simulink model "gm_Prediction_and_cost_function_FCS_MPC_6Phase_PMSM"  (R2022a)
settings: Solver=FixedStepDiscrete  StartTime=0.0  StopTime=10.0  RelTol=1e-3
undefined symbols (not defined in the file or in its folder): f_c, L_d, L_q, L_x, L_y, p, psi_pm, R_ph
libraries: hdlmdlgenlib x6
(part 1 of 2)
settings Model: Creator=Andre Merx  LastModifiedBy=Andre Merx
settings SolverCC: AlgebraicLoopSolver=TrustRegion
settings DataIOCC: LimitDataPoints=on  SaveOutput=off  SaveTime=off
settings OptimizationCC: BlockReduction=off  ConditionallyExecuteInputs=off  DefaultParameterBehavior=Inlined  LifeSpan=inf
settings DebuggingCC: AlgebraicLoopMsg=error  InheritedTsInSrcMsg=none  SingleTaskRateTransMsg=error  UnconnectedInputMsg=warning  UnconnectedOutputMsg=warning  UnconnectedLineMsg=warning  AllowSymbolicDim=off  StrictBusMsg=ErrorOnBusTreatedAsVector  SFUnexpectedBacktrackingDiag=warning  SFNoUnconditionalDefaultTransitionDiag=warning  SFExecutionAtInitializationDiag=none  SFMachineParentedDataDiag=warning  ArithmeticOperatorsInVariantConditions=warning
settings HardwareCC: ProdBitPerPointer=32  ProdBitPerSizeT=32  ProdBitPerPtrDiffT=32  ProdLargestAtomicFloat=None  ProdIntDivRoundTo=Undefined  ProdEndianess=Unspecified  ProdWordSize=32  ProdHWDeviceType=ASIC/FPGA->ASIC/FPGA  ProdEqTarget=off
settings SFSimCC: SimUseLocalCustomCode=off  CustomCodeUndefinedFunction=UseInterfaceOnly
settings RTWCC: RTWUseLocalCustomCode=off
settings CodeAppCC: StateflowObjectComments=on
settings GRTTargetCC: TargetLangStandard=C89/C90 (ANSI)
settings ConfigComp: CovScope=ReferencedModels  CovMetricSettings=dw  CovSaveCumulativeToWorkspaceVar=on  CovSaveSingleToWorkspaceVar=on  CovExternalEMLEnable=off  CovSFcnEnable=off

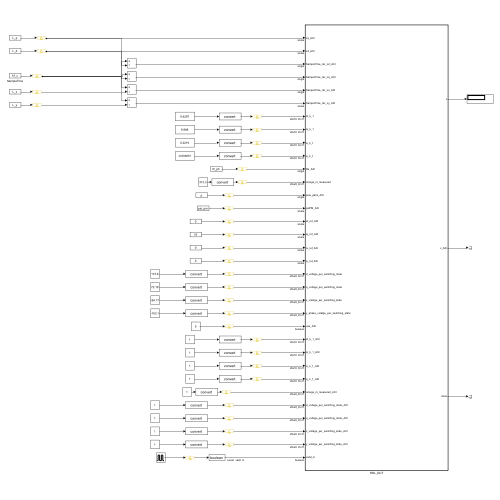
[thumbnail: Simulink's stored preview of the top-level diagram]
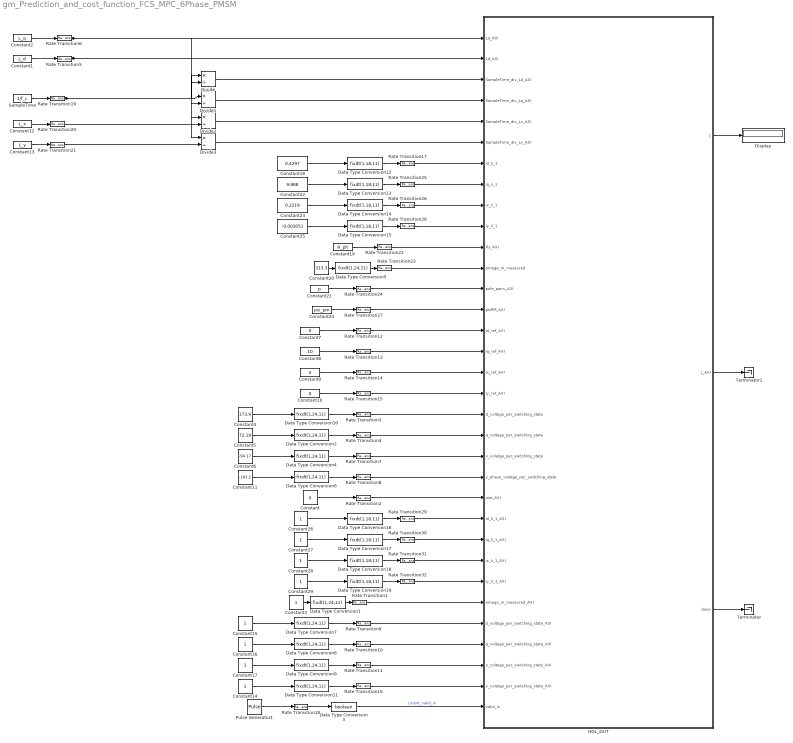
== system gm_Prediction_and_cost_function_FCS_MPC_6Phase_PMSM ==
  Constant : Constant  Value=0  OutDataTypeStr=boolean
  Constant1 : Constant  Value=L_d  OutDataTypeStr=single  SampleTime=-1
  Constant10 : Constant  Value=0  OutDataTypeStr=single  SampleTime=-1
  Constant11 : Constant  Value=-163.1
  Constant12 : Constant  Value=L_x  OutDataTypeStr=single  SampleTime=-1
  Constant13 : Constant  Value=L_y  OutDataTypeStr=single  SampleTime=-1
  Constant{3,14..17,26..29} (9 alike) : Constant
  Constant18 : Constant  Value=0.4297
  Constant19 : Constant  Value=R_ph  OutDataTypeStr=single  SampleTime=-1
  Constant2 : Constant  Value=L_q  OutDataTypeStr=single  SampleTime=-1
  Constant20 : Constant  Value=313.3
  Constant21 : Constant  Value=p  OutDataTypeStr=single  SampleTime=-1
  Constant22 : Constant  Value=9.988
  Constant23 : Constant  Value=0.2219
  Constant24 : Constant  Value=psi_pm  OutDataTypeStr=single  SampleTime=-1
  Constant25 : Constant  Value=-0.003051
  Constant4 : Constant  Value=173.9
  Constant5 : Constant  Value=72.19
  Constant6 : Constant  Value=-94.17
  Constant7 : Constant  Value=0  OutDataTypeStr=single  SampleTime=-1
  Constant8 : Constant  Value=10  OutDataTypeStr=single  SampleTime=-1
  Constant9 : Constant  Value=0  OutDataTypeStr=single  SampleTime=-1
  Data Type Conversion{1..2,4..11} (10 alike) : DataTypeConversion  OutDataTypeStr=fixdt(1,24,11)  SaturateOnIntegerOverflow=off  RndMeth=Floor
  Data Type Conversion{12..19} (8 alike) : DataTypeConversion  OutDataTypeStr=fixdt(1,18,11)  SaturateOnIntegerOverflow=off  RndMeth=Floor
  Data Type Conversion3 : DataTypeConversion  OutDataTypeStr=boolean  SaturateOnIntegerOverflow=off  RndMeth=Floor
  Display : Display
  Divide{,1..3} (4 alike) : Product  Inputs=*/  RndMeth=Zero  SaturateOnIntegerOverflow=on
  HDL_DUT : Subsystem  TreatAsAtomicUnit=on
  Pulse Generator1 : DiscretePulseGenerator  PulseType=Time based  Period=1/f_c
  Rate Transition{1..32} (32 alike) : RateTransition  OutPortSampleTime=Rt
  SampleTime : Constant  Value=1/f_c  OutDataTypeStr=single  SampleTime=-1
  Terminator : Terminator
  Terminator1 : Terminator
  wires:
  Rate Transition31/1 -> HDL_DUT/26(ix_k_1_AXI)
  Rate Transition29/1 -> HDL_DUT/24(id_k_1_AXI)
  Constant27/1 -> Data Type Conversion17/1
  Rate Transition30/1 -> HDL_DUT/25(iq_k_1_AXI)
  Data Type Conversion19/1 -> Rate Transition32/1
  Constant28/1 -> Data Type Conversion18/1
  Data Type Conversion18/1 -> Rate Transition31/1
  Data Type Conversion16/1 -> Rate Transition29/1
  Constant26/1 -> Data Type Conversion16/1
  Constant29/1 -> Data Type Conversion19/1
  Data Type Conversion17/1 -> Rate Transition30/1
  Rate Transition32/1 -> HDL_DUT/27(iy_k_1_AXI)
  Constant25/1 -> Data Type Conversion15/1
  Constant23/1 -> Data Type Conversion14/1
  Constant22/1 -> Data Type Conversion13/1
  Constant18/1 -> Data Type Conversion12/1
  Rate Transition28/1 -> HDL_DUT/10(iy_k_1)
  Data Type Conversion15/1 -> Rate Transition28/1
  Rate Transition26/1 -> HDL_DUT/9(ix_k_1)
  Data Type Conversion14/1 -> Rate Transition26/1
  Rate Transition25/1 -> HDL_DUT/8(iq_k_1)
  Data Type Conversion13/1 -> Rate Transition25/1
  Rate Transition17/1 -> HDL_DUT/7(id_k_1)
  Data Type Conversion12/1 -> Rate Transition17/1
  Rate Transition9/1 -> HDL_DUT/29(d_voltage_per_switching_state_AXI)
  Data Type Conversion7/1 -> Rate Transition9/1
  Data Type Conversion11/1 -> Rate Transition16/1
  Data Type Conversion9/1 -> Rate Transition11/1
  Data Type Conversion8/1 -> Rate Transition10/1
  Rate Transition11/1 -> HDL_DUT/31(x_voltage_per_switching_state_AXI)
  Rate Transition10/1 -> HDL_DUT/30(q_voltage_per_switching_state_AXI)
  Constant16/1 -> Data Type Conversion8/1
  Rate Transition16/1 -> HDL_DUT/32(y_volatge_per_switching_state_AXI)
  Constant14/1 -> Data Type Conversion11/1
  Constant15/1 -> Data Type Conversion7/1
  Constant17/1 -> Data Type Conversion9/1
  Constant11/1 -> Data Type Conversion6/1
  Constant6/1 -> Data Type Conversion4/1
  Constant5/1 -> Data Type Conversion2/1
  Constant4/1 -> Data Type Conversion10/1
  Rate Transition8/1 -> HDL_DUT/22(y_phase_volatge_per_switching_state)
  Data Type Conversion6/1 -> Rate Transition8/1
  Rate Transition7/1 -> HDL_DUT/21(x_volatge_per_switching_state)
  Data Type Conversion4/1 -> Rate Transition7/1
  Rate Transition4/1 -> HDL_DUT/20(q_voltage_per_switching_state)
  Data Type Conversion2/1 -> Rate Transition4/1
  Rate Transition3/1 -> HDL_DUT/19(d_voltage_per_switching_state)
  Data Type Conversion10/1 -> Rate Transition3/1
  Rate Transition2/1 -> HDL_DUT/23(use_AXI)
  Constant/1 -> Rate Transition2/1
  Rate Transition1/1 -> HDL_DUT/28(omega_m_measured_AXI)
  Data Type Conversion1/1 -> Rate Transition1/1
  Constant3/1 -> Data Type Conversion1/1
  Pulse Generator1/1 -> Rate Transition18/1
  Rate Transition18/1 -> Data Type Conversion3/1
  Data Type Conversion3/1 -> HDL_DUT/33(valid_in)  "curent_valid_in"
  HDL_DUT/1(J) -> Display/1
  HDL_DUT/2(J_AXI) -> Terminator1/1
  HDL_DUT/3(done) -> Terminator/1
  Rate Transition15/1 -> HDL_DUT/18(iy_ref_AXI)
  Rate Transition14/1 -> HDL_DUT/17(ix_ref_AXI)
  Rate Transition13/1 -> HDL_DUT/16(iq_ref_AXI)
  Rate Transition12/1 -> HDL_DUT/15(id_ref_AXI)
  Divide3/1 -> HDL_DUT/6(SampleTime_div_Ly_AXI)
  Divide2/1 -> HDL_DUT/5(SampleTime_div_Lx_AXI)
  Divide1/1 -> HDL_DUT/4(SampleTime_div_Lq_AXI)
  Divide/1 -> HDL_DUT/3(SampleTime_div_Ld_AXI)
  SampleTime/1 -> Rate Transition19/1
  Rate Transition20/1 -> Divide2/2
  Rate Transition19/1 -> Divide1/1, Divide/1, Divide2/1, Divide3/1
  Constant12/1 -> Rate Transition20/1
  Constant2/1 -> Rate Transition6/1
  Rate Transition21/1 -> Divide3/2
  Constant13/1 -> Rate Transition21/1
  Constant1/1 -> Rate Transition5/1
  Rate Transition5/1 -> Divide/2, HDL_DUT/2(Ld_AXI)
  Rate Transition6/1 -> Divide1/2, HDL_DUT/1(Lq_AXI)
  Constant19/1 -> Rate Transition22/1
  Constant20/1 -> Data Type Conversion5/1
  Rate Transition22/1 -> HDL_DUT/11(Rs_AXI)
  Rate Transition23/1 -> HDL_DUT/12(omega_m_measured)
  Constant24/1 -> Rate Transition27/1
  Constant21/1 -> Rate Transition24/1
  Data Type Conversion5/1 -> Rate Transition23/1
  Rate Transition27/1 -> HDL_DUT/14(psiPM_AXI)
  Rate Transition24/1 -> HDL_DUT/13(pole_pairs_AXI)
  Constant10/1 -> Rate Transition15/1
  Constant8/1 -> Rate Transition13/1
  Constant9/1 -> Rate Transition14/1
  Constant7/1 -> Rate Transition12/1

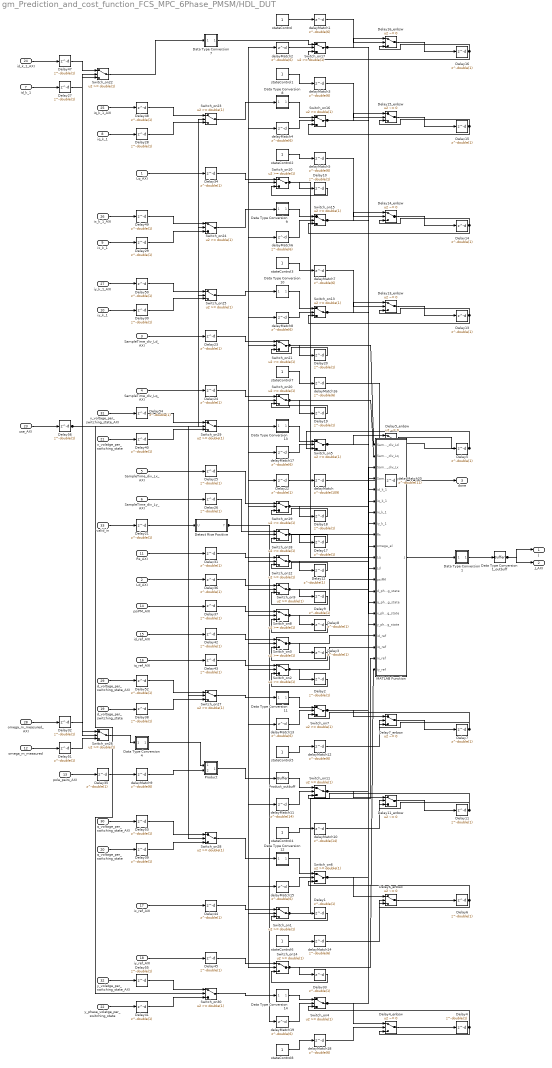
== system gm_Prediction_and_cost_function_FCS_MPC_6Phase_PMSM/HDL_DUT ==
  Lq_AXI : Inport  OutDataTypeStr=single  PortDimensions=1  SampleTime=1e-08
  Ld_AXI : Inport  Port=2  OutDataTypeStr=single  PortDimensions=1  SampleTime=1e-08
  SampleTime_div_Ld_AXI : Inport  Port=3  OutDataTypeStr=single  PortDimensions=1  SampleTime=1e-08
  SampleTime_div_Lq_AXI : Inport  Port=4  OutDataTypeStr=single  PortDimensions=1  SampleTime=1e-08
  SampleTime_div_Lx_AXI : Inport  Port=5  OutDataTypeStr=single  PortDimensions=1  SampleTime=1e-08
  SampleTime_div_Ly_AXI : Inport  Port=6  OutDataTypeStr=single  PortDimensions=1  SampleTime=1e-08
  id_k_1 : Inport  Port=7  OutDataTypeStr=fixdt(1, 18, 11)  PortDimensions=1  SampleTime=1e-08
  iq_k_1 : Inport  Port=8  OutDataTypeStr=fixdt(1, 18, 11)  PortDimensions=1  SampleTime=1e-08
  ix_k_1 : Inport  Port=9  OutDataTypeStr=fixdt(1, 18, 11)  PortDimensions=1  SampleTime=1e-08
  iy_k_1 : Inport  Port=10  OutDataTypeStr=fixdt(1, 18, 11)  PortDimensions=1  SampleTime=1e-08
  Rs_AXI : Inport  Port=11  OutDataTypeStr=single  PortDimensions=1  SampleTime=1e-08
  omega_m_measured : Inport  Port=12  OutDataTypeStr=fixdt(1, 24, 11)  PortDimensions=1  SampleTime=1e-08
  pole_pairs_AXI : Inport  Port=13  OutDataTypeStr=single  PortDimensions=1  SampleTime=1e-08
  psiPM_AXI : Inport  Port=14  OutDataTypeStr=single  PortDimensions=1  SampleTime=1e-08
  id_ref_AXI : Inport  Port=15  OutDataTypeStr=single  PortDimensions=1  SampleTime=1e-08
  iq_ref_AXI : Inport  Port=16  OutDataTypeStr=single  PortDimensions=1  SampleTime=1e-08
  ix_ref_AXI : Inport  Port=17  OutDataTypeStr=single  PortDimensions=1  SampleTime=1e-08
  iy_ref_AXI : Inport  Port=18  OutDataTypeStr=single  PortDimensions=1  SampleTime=1e-08
  d_voltage_per_switching_state : Inport  Port=19  OutDataTypeStr=fixdt(1, 24, 11)  PortDimensions=1  SampleTime=1e-08
  q_voltage_per_switching_state : Inport  Port=20  OutDataTypeStr=fixdt(1, 24, 11)  PortDimensions=1  SampleTime=1e-08
  x_volatge_per_switching_state : Inport  Port=21  OutDataTypeStr=fixdt(1, 24, 11)  PortDimensions=1  SampleTime=1e-08
  y_phase_volatge_per_switching_state : Inport  Port=22  OutDataTypeStr=fixdt(1, 24, 11)  PortDimensions=1  SampleTime=1e-08
  use_AXI : Inport  Port=23  OutDataTypeStr=boolean  PortDimensions=1  SampleTime=1e-08
  id_k_1_AXI : Inport  Port=24  OutDataTypeStr=fixdt(1, 18, 11)  PortDimensions=1  SampleTime=1e-08
  iq_k_1_AXI : Inport  Port=25  OutDataTypeStr=fixdt(1, 18, 11)  PortDimensions=1  SampleTime=1e-08
  ix_k_1_AXI : Inport  Port=26  OutDataTypeStr=fixdt(1, 18, 11)  PortDimensions=1  SampleTime=1e-08
  iy_k_1_AXI : Inport  Port=27  OutDataTypeStr=fixdt(1, 18, 11)  PortDimensions=1  SampleTime=1e-08
  omega_m_measured_AXI : Inport  Port=28  OutDataTypeStr=fixdt(1, 24, 11)  PortDimensions=1  SampleTime=1e-08
  d_voltage_per_switching_state_AXI : Inport  Port=29  OutDataTypeStr=fixdt(1, 24, 11)  PortDimensions=1  SampleTime=1e-08
  q_voltage_per_switching_state_AXI : Inport  Port=30  OutDataTypeStr=fixdt(1, 24, 11)  PortDimensions=1  SampleTime=1e-08
  x_voltage_per_switching_state_AXI : Inport  Port=31  OutDataTypeStr=fixdt(1, 24, 11)  PortDimensions=1  SampleTime=1e-08
  y_volatge_per_switching_state_AXI : Inport  Port=32  OutDataTypeStr=fixdt(1, 24, 11)  PortDimensions=1  SampleTime=1e-08
  valid_in : Inport  Port=33  OutDataTypeStr=boolean  PortDimensions=1  SampleTime=1e-08
  Data Type Conversion1 : Subsystem
      mask Display: disp('NFP\nconv');
  Data Type Conversion10 : Subsystem
      mask Display: disp('NFP\nconv');
  Data Type Conversion11 : Subsystem
      mask Display: disp('NFP\nconv');
  Data Type Conversion12 : Subsystem
      mask Display: disp('NFP\nconv');
  Data Type Conversion13 : Subsystem
      mask Display: disp('NFP\nconv');
  Data Type Conversion14 : Subsystem
      mask Display: disp('NFP\nconv');
  Data Type Conversion1_outbuff : hdlmdlgenlib/Buffer
      settings: SourceProductBaseCode=SL
  Data Type Conversion4 : Subsystem
      mask Display: disp('NFP\nconv');
  Data Type Conversion7 : Subsystem
      mask Display: disp('NFP\nconv');
  Data Type Conversion8 : Subsystem
      mask Display: disp('NFP\nconv');
  Data Type Conversion9 : Subsystem
      mask Display: disp('NFP\nconv');
  Delay{1..45,47..56} (55 alike) : Delay  DelayLength=double(1)  InitialCondition=0  SampleTime=1e-08
  Delay11_enbsw : Switch  Criteria=u2 ~= 0  Threshold=double(0)  OutDataTypeStr=single  SampleTime=1e-08  SaturateOnIntegerOverflow=off  InputSameDT=off
  Delay13_enbsw : Switch  Criteria=u2 ~= 0  Threshold=double(0)  OutDataTypeStr=single  SampleTime=1e-08  SaturateOnIntegerOverflow=off  InputSameDT=off
  Delay14_enbsw : Switch  Criteria=u2 ~= 0  Threshold=double(0)  OutDataTypeStr=single  SampleTime=1e-08  SaturateOnIntegerOverflow=off  InputSameDT=off
  Delay15_enbsw : Switch  Criteria=u2 ~= 0  Threshold=double(0)  OutDataTypeStr=single  SampleTime=1e-08  SaturateOnIntegerOverflow=off  InputSameDT=off
  Delay16_enbsw : Switch  Criteria=u2 ~= 0  Threshold=double(0)  OutDataTypeStr=single  SampleTime=1e-08  SaturateOnIntegerOverflow=off  InputSameDT=off
  Delay4_enbsw : Switch  Criteria=u2 ~= 0  Threshold=double(0)  OutDataTypeStr=single  SampleTime=1e-08  SaturateOnIntegerOverflow=off  InputSameDT=off
  Delay5_enbsw : Switch  Criteria=u2 ~= 0  Threshold=double(0)  OutDataTypeStr=single  SampleTime=1e-08  SaturateOnIntegerOverflow=off  InputSameDT=off
  Delay6_enbsw : Switch  Criteria=u2 ~= 0  Threshold=double(0)  OutDataTypeStr=single  SampleTime=1e-08  SaturateOnIntegerOverflow=off  InputSameDT=off
  Delay7_enbsw : Switch  Criteria=u2 ~= 0  Threshold=double(0)  OutDataTypeStr=single  SampleTime=1e-08  SaturateOnIntegerOverflow=off  InputSameDT=off
  Detect Rise Positive : Subsystem  mask(Detect Rise Positive){vinit=double(0), InputProcessing=Elements as channels (sample based), OutDataTypeStr=boolean}
      mask prompts: vinit "Simulink:masks:InitialCondition_MP"; InputProcessing "Simulink:masks:InputProcessing_MP"; OutDataTypeStr "Simulink:masks:OutputDataType_MP"
      mask help: Simulink:masks:DetectRisePositive_MD
      mask init:
      | InputProcessing = 'Elements as channels (sample based)';
      | OutDataTypeStr = 'boolean';
      | vinit = double(0);
      mask TypeOptions InputProcessing: Simulink:masks:ColumnsAsChannelsFrameBased | Simulink:masks:ElementsAsChannelsSampleBased
      mask TypeOptions OutDataTypeStr: Simulink:masks:uint8 | Simulink:masks:boolean
      mask Display: fprintf('U > 0\n&  NOT\nU/z > 0')
  MATLAB Function : Subsystem
  Product : Subsystem
      mask Display: disp('NFP\nmul');
  Product_outbuff : hdlmdlgenlib/Buffer
      settings: SourceProductBaseCode=SL
  Switch_on{1..21} (21 alike) : Switch  Threshold=double(1)  OutDataTypeStr=single  RndMeth=Simplest  SampleTime=1e-08  SaturateOnIntegerOverflow=off  InputSameDT=off
  Switch_on{22..25} (4 alike) : Switch  Threshold=double(1)  OutDataTypeStr=fixdt(1, 18, 11)  RndMeth=Simplest  SampleTime=1e-08  SaturateOnIntegerOverflow=off  InputSameDT=off
  Switch_on{26..30} (5 alike) : Switch  Threshold=double(1)  OutDataTypeStr=fixdt(1, 24, 11)  RndMeth=Simplest  SampleTime=1e-08  SaturateOnIntegerOverflow=off  InputSameDT=off
  delayMatch : Delay  DelayLength=double(109)  InitialCondition=0  SampleTime=1e-08
  delayMatch{1..9,12..19} (17 alike) : Delay  DelayLength=double(6)  InitialCondition=0  SampleTime=1e-08
  delayMatch10 : Delay  DelayLength=double(14)  InitialCondition=0  SampleTime=1e-08
  delayMatch11 : Delay  DelayLength=double(14)  InitialCondition=0  SampleTime=1e-08
  delayMatch20 : Delay  DelayLength=double(11)  InitialCondition=0  SampleTime=1e-08
  stateControl{,1..8} (9 alike) : Constant  OutDataTypeStr=boolean  SampleTime=1e-08
  J : Outport  SampleTime=1e-08
  J_AXI : Outport  Port=2  SampleTime=1e-08
  done : Outport  Port=3  SampleTime=1e-08
  wires:
  Lq_AXI/1 -> Delay34/1
  Ld_AXI/1 -> Delay36/1
  SampleTime_div_Ld_AXI/1 -> Delay23/1
  SampleTime_div_Lq_AXI/1 -> Delay24/1
  SampleTime_div_Lx_AXI/1 -> Delay25/1
  SampleTime_div_Ly_AXI/1 -> Delay26/1
  id_k_1/1 -> Delay27/1
  iq_k_1/1 -> Delay28/1
  ix_k_1/1 -> Delay29/1
  iy_k_1/1 -> Delay30/1
  Rs_AXI/1 -> Delay31/1
  omega_m_measured/1 -> Delay51/1
  pole_pairs_AXI/1 -> Delay35/1
  psiPM_AXI/1 -> Delay37/1
  id_ref_AXI/1 -> Delay42/1
  iq_ref_AXI/1 -> Delay43/1
  ix_ref_AXI/1 -> Delay44/1
  iy_ref_AXI/1 -> Delay45/1
  d_voltage_per_switching_state/1 -> Delay38/1
  q_voltage_per_switching_state/1 -> Delay39/1
  x_volatge_per_switching_state/1 -> Delay40/1
  y_phase_volatge_per_switching_state/1 -> Delay41/1
  use_AXI/1 -> Delay56/1
  id_k_1_AXI/1 -> Delay47/1
  iq_k_1_AXI/1 -> Delay48/1
  ix_k_1_AXI/1 -> Delay49/1
  iy_k_1_AXI/1 -> Delay50/1
  omega_m_measured_AXI/1 -> Delay32/1
  d_voltage_per_switching_state_AXI/1 -> Delay52/1
  q_voltage_per_switching_state_AXI/1 -> Delay53/1
  x_voltage_per_switching_state_AXI/1 -> Delay54/1
  y_volatge_per_switching_state_AXI/1 -> Delay55/1
  valid_in/1 -> Delay21/1
  Data Type Conversion1_outbuff/1 -> J_AXI/1, J/1
  Delay21/1 -> Detect Rise Positive/1(U)
  delayMatch20/1 -> done/1
  Delay23/1 -> Switch_on21/1
  Delay24/1 -> Switch_on20/1
  Delay25/1 -> Switch_on19/1
  Delay26/1 -> Switch_on18/1
  Delay27/1 -> Switch_on22/3
  Delay28/1 -> Switch_on23/3
  Delay29/1 -> Switch_on24/3
  Delay30/1 -> Switch_on25/3
  Delay31/1 -> Switch_on12/1
  Delay32/1 -> Switch_on26/1
  Delay34/1 -> Switch_on10/1
  delayMatch9/1 -> Product/2(In2)
  Delay36/1 -> Switch_on9/1
  Delay37/1 -> Switch_on8/1
  Delay38/1 -> Switch_on27/3
  Delay39/1 -> Switch_on28/3
  Delay40/1 -> Switch_on29/3
  Delay41/1 -> Switch_on30/3
  Delay42/1 -> Switch_on3/1
  Delay43/1 -> Switch_on2/1
  Delay44/1 -> Switch_on1/1
  Delay45/1 -> Switch_on14/1
  Delay47/1 -> Switch_on22/1
  Delay48/1 -> Switch_on23/1
  Delay49/1 -> Switch_on24/1
  Delay50/1 -> Switch_on25/1
  Delay51/1 -> Switch_on26/3
  Delay52/1 -> Switch_on27/1
  Delay53/1 -> Switch_on28/1
  Delay54/1 -> Switch_on29/1
  Delay55/1 -> Switch_on30/1
  Delay56/1 -> Switch_on30/2, Switch_on29/2, Switch_on28/2, Switch_on27/2, Switch_on26/2, Switch_on25/2, Switch_on24/2, Switch_on23/2, Switch_on22/2
  delayMatch2/1 -> Switch_on17/2
  MATLAB Function/1(J) -> Data Type Conversion1/1(In1)
  Product_outbuff/1 -> Switch_on11/1
  Switch_on1/1 -> MATLAB Function/20(ix_ref), Delay1/1
  Switch_on10/1 -> MATLAB Function/11(Lq), Delay10/1
  Switch_on12/1 -> MATLAB Function/9(Rs), Delay12/1
  Switch_on14/1 -> MATLAB Function/21(iy_ref), Delay33/1
  Switch_on18/1 -> MATLAB Function/4(SampleTime_div_Ly), Delay17/1
  Switch_on19/1 -> MATLAB Function/3(SampleTime_div_Lx), Delay18/1
  Switch_on2/1 -> MATLAB Function/19(iq_ref), Delay2/1
  Switch_on20/1 -> MATLAB Function/2(SampleTime_div_Lq), Delay19/1
  Switch_on21/1 -> MATLAB Function/1(SampleTime_div_Ld), Delay20/1
  Switch_on22/1 -> Data Type Conversion7/1(In1)
  Switch_on23/1 -> Data Type Conversion8/1(In1)
  Switch_on24/1 -> Data Type Conversion9/1(In1)
  Switch_on25/1 -> Data Type Conversion10/1(In1)
  Switch_on26/1 -> Data Type Conversion4/1(In1)
  Switch_on27/1 -> Data Type Conversion11/1(In1)
  Switch_on28/1 -> Data Type Conversion12/1(In1)
  Switch_on29/1 -> Data Type Conversion13/1(In1)
  Switch_on3/1 -> MATLAB Function/18(id_ref), Delay3/1
  Switch_on30/1 -> Data Type Conversion14/1(In1)
  Switch_on8/1 -> MATLAB Function/13(psiPM), Delay8/1
  Switch_on9/1 -> MATLAB Function/12(Ld), Delay9/1
  Delay22/1 -> delayMatch/1
  Data Type Conversion1/1(Out1) -> Data Type Conversion1_outbuff/1
  Data Type Conversion10/1(Out1) -> Switch_on13/1
  Data Type Conversion11/1(Out1) -> Switch_on7/1
  Data Type Conversion12/1(Out1) -> Switch_on6/1
  Data Type Conversion13/1(Out1) -> Switch_on5/1
  Data Type Conversion14/1(Out1) -> Switch_on4/1
  Data Type Conversion4/1(Out1) -> Product/1(In1)
  Data Type Conversion7/1(Out1) -> Switch_on17/1
  Data Type Conversion8/1(Out1) -> Switch_on16/1
  Data Type Conversion9/1(Out1) -> Switch_on15/1
  Product/1(Out1) -> Product_outbuff/1
  delayMatch1/1 -> Delay16_enbsw/2
  delayMatch3/1 -> Delay15_enbsw/2
  delayMatch5/1 -> Delay14_enbsw/2
  delayMatch7/1 -> Delay13_enbsw/2
  delayMatch10/1 -> Delay11_enbsw/2
  delayMatch12/1 -> Delay7_enbsw/2
  delayMatch14/1 -> Delay6_enbsw/2
  delayMatch16/1 -> Delay5_enbsw/2
  delayMatch18/1 -> Delay4_enbsw/2
  stateControl/1 -> delayMatch1/1
  delayMatch4/1 -> Switch_on16/2
  stateControl1/1 -> delayMatch3/1
  delayMatch6/1 -> Switch_on15/2
  stateControl2/1 -> delayMatch5/1
  delayMatch8/1 -> Switch_on13/2
  stateControl3/1 -> delayMatch7/1
  delayMatch11/1 -> Switch_on11/2
  Delay35/1 -> delayMatch9/1
  stateControl4/1 -> delayMatch10/1
  delayMatch13/1 -> Switch_on7/2
  stateControl5/1 -> delayMatch12/1
  delayMatch15/1 -> Switch_on6/2
  stateControl6/1 -> delayMatch14/1
  delayMatch17/1 -> Switch_on5/2
  stateControl7/1 -> delayMatch16/1
  delayMatch19/1 -> Switch_on4/2
  stateControl8/1 -> delayMatch18/1
  Detect Rise Positive/1(Y) -> delayMatch19/1, delayMatch17/1, delayMatch15/1, delayMatch13/1, delayMatch11/1, delayMatch8/1, delayMatch6/1, delayMatch4/1, delayMatch2/1, Delay22/1, Switch_on21/2, Switch_on20/2, Switch_on19/2, Switch_on18/2, Switch_on12/2, Switch_on10/2, Switch_on9/2, Switch_on8/2, Switch_on3/2, Switch_on2/2, Switch_on1/2, Switch_on14/2
  delayMatch/1 -> delayMatch20/1
  Switch_on17/1 -> MATLAB Function/5(id_k_1), Delay16_enbsw/1
  Switch_on16/1 -> MATLAB Function/6(iq_k_1), Delay15_enbsw/1
  Switch_on15/1 -> MATLAB Function/7(ix_k_1), Delay14_enbsw/1
  Switch_on13/1 -> MATLAB Function/8(iy_k_1), Delay13_enbsw/1
  Switch_on11/1 -> MATLAB Function/10(omega_el), Delay11_enbsw/1
  Switch_on7/1 -> MATLAB Function/14(d_phase_voltage_per_switching_state), Delay7_enbsw/1
  Switch_on6/1 -> MATLAB Function/15(q_phase_voltage_per_switching_state), Delay6_enbsw/1
  Switch_on5/1 -> MATLAB Function/16(x_phase_voltage_per_switching_state), Delay5_enbsw/1
  Switch_on4/1 -> MATLAB Function/17(y_phase_voltage_per_switching_state), Delay4_enbsw/1
  Delay20/1 -> Switch_on21/3
  Delay19/1 -> Switch_on20/3
  Delay18/1 -> Switch_on19/3
  Delay17/1 -> Switch_on18/3
  Delay16_enbsw/1 -> Delay16/1
  Delay16/1 -> Switch_on17/3, Delay16_enbsw/3
  Delay15_enbsw/1 -> Delay15/1
  Delay15/1 -> Switch_on16/3, Delay15_enbsw/3
  Delay14_enbsw/1 -> Delay14/1
  Delay14/1 -> Switch_on15/3, Delay14_enbsw/3
  Delay13_enbsw/1 -> Delay13/1
  Delay13/1 -> Switch_on13/3, Delay13_enbsw/3
  Delay12/1 -> Switch_on12/3
  Delay11_enbsw/1 -> Delay11/1
  Delay11/1 -> Switch_on11/3, Delay11_enbsw/3
  Delay10/1 -> Switch_on10/3
  Delay9/1 -> Switch_on9/3
  Delay8/1 -> Switch_on8/3
  Delay7_enbsw/1 -> Delay7/1
  Delay7/1 -> Switch_on7/3, Delay7_enbsw/3
  Delay6_enbsw/1 -> Delay6/1
  Delay6/1 -> Switch_on6/3, Delay6_enbsw/3
  Delay5_enbsw/1 -> Delay5/1
  Delay5/1 -> Switch_on5/3, Delay5_enbsw/3
  Delay4_enbsw/1 -> Delay4/1
  Delay4/1 -> Switch_on4/3, Delay4_enbsw/3
  Delay3/1 -> Switch_on3/3
  Delay2/1 -> Switch_on2/3
  Delay1/1 -> Switch_on1/3
  Delay33/1 -> Switch_on14/3

== system gm_Prediction_and_cost_function_FCS_MPC_6Phase_PMSM/HDL_DUT/Data Type Conversion1 ==
  In1 : Inport
  Data Type Conversion1 : DataTypeConversion  OutDataTypeStr=fixdt(1, 20, 11)  RndMeth=Nearest  SampleTime=1e-08  SaturateOnIntegerOverflow=off
  Data Type Conversion1_pd1 : Delay  DelayLength=6
  Out1 : Outport
  wires:
  In1/1 -> Data Type Conversion1/1
  Data Type Conversion1/1 -> Data Type Conversion1_pd1/1
  Data Type Conversion1_pd1/1 -> Out1/1

== system gm_Prediction_and_cost_function_FCS_MPC_6Phase_PMSM/HDL_DUT/Data Type Conversion10 ==
  In1 : Inport
  Data Type Conversion10 : DataTypeConversion  OutDataTypeStr=single  RndMeth=Nearest  SampleTime=1e-08  SaturateOnIntegerOverflow=off
  Data Type Conversion10_pd1 : Delay  DelayLength=6
  Out1 : Outport
  wires:
  In1/1 -> Data Type Conversion10/1
  Data Type Conversion10/1 -> Data Type Conversion10_pd1/1
  Data Type Conversion10_pd1/1 -> Out1/1

== system gm_Prediction_and_cost_function_FCS_MPC_6Phase_PMSM/HDL_DUT/Data Type Conversion11 ==
  In1 : Inport
  Data Type Conversion11 : DataTypeConversion  OutDataTypeStr=single  RndMeth=Nearest  SampleTime=1e-08  SaturateOnIntegerOverflow=off
  Data Type Conversion11_pd1 : Delay  DelayLength=6
  Out1 : Outport
  wires:
  In1/1 -> Data Type Conversion11/1
  Data Type Conversion11/1 -> Data Type Conversion11_pd1/1
  Data Type Conversion11_pd1/1 -> Out1/1

== system gm_Prediction_and_cost_function_FCS_MPC_6Phase_PMSM/HDL_DUT/Data Type Conversion12 ==
  In1 : Inport
  Data Type Conversion12 : DataTypeConversion  OutDataTypeStr=single  RndMeth=Nearest  SampleTime=1e-08  SaturateOnIntegerOverflow=off
  Data Type Conversion12_pd1 : Delay  DelayLength=6
  Out1 : Outport
  wires:
  In1/1 -> Data Type Conversion12/1
  Data Type Conversion12/1 -> Data Type Conversion12_pd1/1
  Data Type Conversion12_pd1/1 -> Out1/1

== system gm_Prediction_and_cost_function_FCS_MPC_6Phase_PMSM/HDL_DUT/Data Type Conversion13 ==
  In1 : Inport
  Data Type Conversion13 : DataTypeConversion  OutDataTypeStr=single  RndMeth=Nearest  SampleTime=1e-08  SaturateOnIntegerOverflow=off
  Data Type Conversion13_pd1 : Delay  DelayLength=6
  Out1 : Outport
  wires:
  In1/1 -> Data Type Conversion13/1
  Data Type Conversion13/1 -> Data Type Conversion13_pd1/1
  Data Type Conversion13_pd1/1 -> Out1/1

== system gm_Prediction_and_cost_function_FCS_MPC_6Phase_PMSM/HDL_DUT/Data Type Conversion14 ==
  In1 : Inport
  Data Type Conversion14 : DataTypeConversion  OutDataTypeStr=single  RndMeth=Nearest  SampleTime=1e-08  SaturateOnIntegerOverflow=off
  Data Type Conversion14_pd1 : Delay  DelayLength=6
  Out1 : Outport
  wires:
  In1/1 -> Data Type Conversion14/1
  Data Type Conversion14/1 -> Data Type Conversion14_pd1/1
  Data Type Conversion14_pd1/1 -> Out1/1

== system gm_Prediction_and_cost_function_FCS_MPC_6Phase_PMSM/HDL_DUT/Data Type Conversion4 ==
  In1 : Inport
  Data Type Conversion4 : DataTypeConversion  OutDataTypeStr=single  RndMeth=Nearest  SampleTime=1e-08  SaturateOnIntegerOverflow=off
  Data Type Conversion4_pd1 : Delay  DelayLength=6
  Out1 : Outport
  wires:
  In1/1 -> Data Type Conversion4/1
  Data Type Conversion4/1 -> Data Type Conversion4_pd1/1
  Data Type Conversion4_pd1/1 -> Out1/1

== system gm_Prediction_and_cost_function_FCS_MPC_6Phase_PMSM/HDL_DUT/Data Type Conversion7 ==
  In1 : Inport
  Data Type Conversion7 : DataTypeConversion  OutDataTypeStr=single  RndMeth=Nearest  SampleTime=1e-08  SaturateOnIntegerOverflow=off
  Data Type Conversion7_pd1 : Delay  DelayLength=6
  Out1 : Outport
  wires:
  In1/1 -> Data Type Conversion7/1
  Data Type Conversion7/1 -> Data Type Conversion7_pd1/1
  Data Type Conversion7_pd1/1 -> Out1/1

== system gm_Prediction_and_cost_function_FCS_MPC_6Phase_PMSM/HDL_DUT/Data Type Conversion8 ==
  In1 : Inport
  Data Type Conversion8 : DataTypeConversion  OutDataTypeStr=single  RndMeth=Nearest  SampleTime=1e-08  SaturateOnIntegerOverflow=off
  Data Type Conversion8_pd1 : Delay  DelayLength=6
  Out1 : Outport
  wires:
  In1/1 -> Data Type Conversion8/1
  Data Type Conversion8/1 -> Data Type Conversion8_pd1/1
  Data Type Conversion8_pd1/1 -> Out1/1

== system gm_Prediction_and_cost_function_FCS_MPC_6Phase_PMSM/HDL_DUT/Data Type Conversion9 ==
  In1 : Inport
  Data Type Conversion9 : DataTypeConversion  OutDataTypeStr=single  RndMeth=Nearest  SampleTime=1e-08  SaturateOnIntegerOverflow=off
  Data Type Conversion9_pd1 : Delay  DelayLength=6
  Out1 : Outport
  wires:
  In1/1 -> Data Type Conversion9/1
  Data Type Conversion9/1 -> Data Type Conversion9_pd1/1
  Data Type Conversion9_pd1/1 -> Out1/1

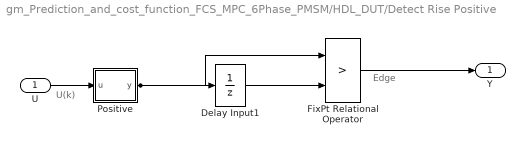
== system gm_Prediction_and_cost_function_FCS_MPC_6Phase_PMSM/HDL_DUT/Detect Rise Positive ==
  note: Edge
  note: U(k)
  U : Inport  OutDataTypeStr=boolean  SampleTime=1e-08
  Delay Input1 : UnitDelay  Description=Store in Global RAM  DisableCoverage=on  InitialCondition=vinit  SampleTime=-1  HasFrameUpgradeWarning=on
  FixPt Relational Operator : RelationalOperator  Operator=>  OutDataTypeStr=boolean  ZeroCross=off  InputSameDT=off
  Positive : Subsystem  mask(Compare To Zero){relop=>, OutDataTypeStr=boolean, ZeroCross=off}
      mask prompts: relop "Simulink:masks:Operator_MP"; OutDataTypeStr "Simulink:masks:OutputDataType_MP"; ZeroCross "Simulink:masks:EnableZerocrossingDetection_MP"
      mask help: Simulink:masks:CompareToZero_MD
      mask init:
      | OutDataTypeStr = 'boolean';
      | ZeroCross = 'off';
      | blkName = 'Prediction_and_cost_function_FCS_MPC_6Phase_PMSM/HDL_DUT/Detect Rise\nPositive/Positive';
      | relop = '>';
      | setValue = 'boolean';
      mask TypeOptions relop: == | ~= | < | <= | >= | >
      mask TypeOptions OutDataTypeStr: Simulink:masks:uint8 | Simulink:masks:boolean
      mask Callback ZeroCross: sl('zeroCrossEnable', gcbh);
      mask Display: disp([relop,' 0'])
  Y : Outport  SampleTime=1e-08
  wires:
  Delay Input1/1 -> FixPt Relational Operator/2
  FixPt Relational Operator/1 -> Y/1
  Positive/1(y) -> FixPt Relational Operator/1, Delay Input1/1
  U/1 -> Positive/1(u)

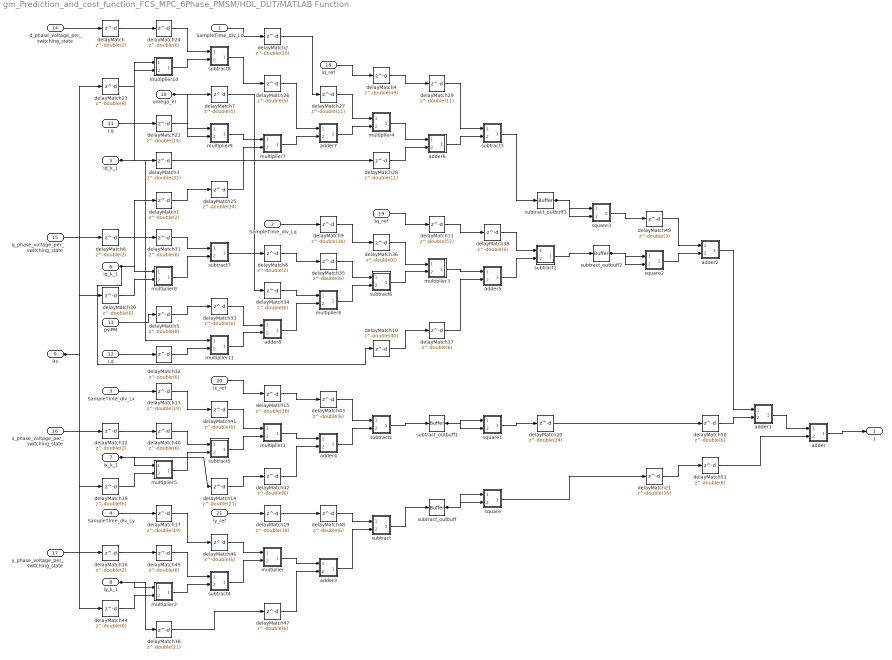
== system gm_Prediction_and_cost_function_FCS_MPC_6Phase_PMSM/HDL_DUT/MATLAB Function ==
  SampleTime_div_Ld : Inport  OutDataTypeStr=single  PortDimensions=1  SampleTime=1e-08
  SampleTime_div_Lq : Inport  Port=2  OutDataTypeStr=single  PortDimensions=1  SampleTime=1e-08
  SampleTime_div_Lx : Inport  Port=3  OutDataTypeStr=single  PortDimensions=1  SampleTime=1e-08
  SampleTime_div_Ly : Inport  Port=4  OutDataTypeStr=single  PortDimensions=1  SampleTime=1e-08
  id_k_1 : Inport  Port=5  OutDataTypeStr=single  PortDimensions=1  SampleTime=1e-08
  iq_k_1 : Inport  Port=6  OutDataTypeStr=single  PortDimensions=1  SampleTime=1e-08
  ix_k_1 : Inport  Port=7  OutDataTypeStr=single  PortDimensions=1  SampleTime=1e-08
  iy_k_1 : Inport  Port=8  OutDataTypeStr=single  PortDimensions=1  SampleTime=1e-08
  Rs : Inport  Port=9  OutDataTypeStr=single  PortDimensions=1  SampleTime=1e-08
  omega_el : Inport  Port=10  OutDataTypeStr=single  PortDimensions=1  SampleTime=1e-08
  Lq : Inport  Port=11  OutDataTypeStr=single  PortDimensions=1  SampleTime=1e-08
  Ld : Inport  Port=12  OutDataTypeStr=single  PortDimensions=1  SampleTime=1e-08
  psiPM : Inport  Port=13  OutDataTypeStr=single  PortDimensions=1  SampleTime=1e-08
  d_phase_voltage_per_switching_state : Inport  Port=14  OutDataTypeStr=single  PortDimensions=1  SampleTime=1e-08
  q_phase_voltage_per_switching_state : Inport  Port=15  OutDataTypeStr=single  PortDimensions=1  SampleTime=1e-08
  x_phase_voltage_per_switching_state : Inport  Port=16  OutDataTypeStr=single  PortDimensions=1  SampleTime=1e-08
  y_phase_voltage_per_switching_state : Inport  Port=17  OutDataTypeStr=single  PortDimensions=1  SampleTime=1e-08
  id_ref : Inport  Port=18  OutDataTypeStr=single  PortDimensions=1  SampleTime=1e-08
  iq_ref : Inport  Port=19  OutDataTypeStr=single  PortDimensions=1  SampleTime=1e-08
  ix_ref : Inport  Port=20  OutDataTypeStr=single  PortDimensions=1  SampleTime=1e-08
  iy_ref : Inport  Port=21  OutDataTypeStr=single  PortDimensions=1  SampleTime=1e-08
  adder : Subsystem
      mask Display: disp('NFP\nadd');
  adder1 : Subsystem
      mask Display: disp('NFP\nadd');
  adder2 : Subsystem
      mask Display: disp('NFP\nadd');
  adder3 : Subsystem
      mask Display: disp('NFP\nadd');
  adder4 : Subsystem
      mask Display: disp('NFP\nadd');
  adder5 : Subsystem
      mask Display: disp('NFP\nadd');
  adder6 : Subsystem
      mask Display: disp('NFP\nadd');
  adder7 : Subsystem
      mask Display: disp('NFP\nadd');
  adder8 : Subsystem
      mask Display: disp('NFP\nadd');
  delayMatch{,1,6,8,12,16} (6 alike) : Delay  DelayLength=double(2)  InitialCondition=0  SampleTime=1e-08
  delayMatch10 : Delay  DelayLength=double(40)  InitialCondition=0  SampleTime=1e-08
  delayMatch11 : Delay  DelayLength=double(57)  InitialCondition=0  SampleTime=1e-08
  delayMatch13 : Delay  DelayLength=double(19)  InitialCondition=0  SampleTime=1e-08
  delayMatch14 : Delay  DelayLength=double(21)  InitialCondition=0  SampleTime=1e-08
  delayMatch15 : Delay  DelayLength=double(38)  InitialCondition=0  SampleTime=1e-08
  delayMatch17 : Delay  DelayLength=double(19)  InitialCondition=0  SampleTime=1e-08
  delayMatch18 : Delay  DelayLength=double(21)  InitialCondition=0  SampleTime=1e-08
  delayMatch19 : Delay  DelayLength=double(38)  InitialCondition=0  SampleTime=1e-08
  delayMatch2 : Delay  DelayLength=double(30)  InitialCondition=0  SampleTime=1e-08
  delayMatch20 : Delay  DelayLength=double(24)  InitialCondition=0  SampleTime=1e-08
  delayMatch21 : Delay  DelayLength=double(35)  InitialCondition=0  SampleTime=1e-08
  delayMatch22 : Delay  DelayLength=double(14)  InitialCondition=0  SampleTime=1e-08
  delayMatch{23..24,30..48,50..51} (23 alike) : Delay  DelayLength=double(6)  InitialCondition=0  SampleTime=1e-08
  delayMatch25 : Delay  DelayLength=double(14)  InitialCondition=0  SampleTime=1e-08
  delayMatch26 : Delay  DelayLength=double(5)  InitialCondition=0  SampleTime=1e-08
  delayMatch27 : Delay  DelayLength=double(11)  InitialCondition=0  SampleTime=1e-08
  delayMatch28 : Delay  DelayLength=double(11)  InitialCondition=0  SampleTime=1e-08
  delayMatch29 : Delay  DelayLength=double(11)  InitialCondition=0  SampleTime=1e-08
  delayMatch3 : Delay  DelayLength=double(32)  InitialCondition=0  SampleTime=1e-08
  delayMatch4 : Delay  DelayLength=double(49)  InitialCondition=0  SampleTime=1e-08
  delayMatch49 : Delay  DelayLength=double(3)  InitialCondition=0  SampleTime=1e-08
  delayMatch5 : Delay  DelayLength=double(8)  InitialCondition=0  SampleTime=1e-08
  delayMatch7 : Delay  DelayLength=double(5)  InitialCondition=0  SampleTime=1e-08
  delayMatch9 : Delay  DelayLength=double(38)  InitialCondition=0  SampleTime=1e-08
  multiplier : Subsystem
      mask Display: disp('NFP\nmul');
  multiplier1 : Subsystem
      mask Display: disp('NFP\nmul');
  multiplier10 : Subsystem
      mask Display: disp('NFP\nmul');
  multiplier11 : Subsystem
      mask Display: disp('NFP\nmul');
  multiplier2 : Subsystem
      mask Display: disp('NFP\nmul');
  multiplier3 : Subsystem
      mask Display: disp('NFP\nmul');
  multiplier4 : Subsystem
      mask Display: disp('NFP\nmul');
  multiplier5 : Subsystem
      mask Display: disp('NFP\nmul');
  multiplier6 : Subsystem
      mask Display: disp('NFP\nmul');
  multiplier7 : Subsystem
      mask Display: disp('NFP\nmul');
  multiplier8 : Subsystem
      mask Display: disp('NFP\nmul');
  multiplier9 : Subsystem
      mask Display: disp('NFP\nmul');
  square : Subsystem
      mask Display: disp('NFP\nmul');
  square1 : Subsystem
      mask Display: disp('NFP\nmul');
  square2 : Subsystem
      mask Display: disp('NFP\nmul');
  square3 : Subsystem
      mask Display: disp('NFP\nmul');
  subtract : Subsystem
      mask Display: disp('NFP\nadd');
  subtract1 : Subsystem
      mask Display: disp('NFP\nadd');
  subtract2 : Subsystem
      mask Display: disp('NFP\nadd');
  subtract3 : Subsystem
      mask Display: disp('NFP\nadd');
  subtract4 : Subsystem
      mask Display: disp('NFP\nadd');
  subtract5 : Subsystem
      mask Display: disp('NFP\nadd');
  subtract6 : Subsystem
      mask Display: disp('NFP\nadd');
  subtract7 : Subsystem
      mask Display: disp('NFP\nadd');
  subtract8 : Subsystem
      mask Display: disp('NFP\nadd');
  subtract_outbuff{,1..3} (4 alike) : hdlmdlgenlib/Buffer
      settings: SourceProductBaseCode=SL
  J : Outport  SampleTime=1e-08  VectorParamsAs1DForOutWhenUnconnected=off
  wires:
  delayMatch27/1 -> multiplier4/1(In1)
  delayMatch36/1 -> multiplier3/1(In1)
  delayMatch41/1 -> multiplier1/1(In1)
  delayMatch46/1 -> multiplier/1(In1)
  delayMatch28/1 -> adder6/2(In2)
  delayMatch25/1 -> multiplier7/2(In2)
  delayMatch42/1 -> adder4/2(In2)
  delayMatch47/1 -> adder3/2(In2)
  delayMatch34/1 -> multiplier6/1(In1)
  delayMatch33/1 -> adder8/1(In1)
  delayMatch24/1 -> subtract8/1(In1)
  delayMatch31/1 -> subtract7/1(In1)
  delayMatch40/1 -> subtract5/1(In1)
  delayMatch45/1 -> subtract4/1(In1)
  delayMatch29/1 -> subtract3/1(In1)
  delayMatch38/1 -> subtract2/1(In1)
  delayMatch43/1 -> subtract1/1(In1)
  delayMatch48/1 -> subtract/1(In1)
  delayMatch51/1 -> adder/2(In2)
  subtract_outbuff/1 -> square/2(In2), square/1(In1)
  delayMatch50/1 -> adder1/2(In2)
  subtract_outbuff1/1 -> square1/2(In2), square1/1(In1)
  delayMatch49/1 -> adder2/1(In1)
  subtract_outbuff2/1 -> square2/2(In2), square2/1(In1)
  subtract_outbuff3/1 -> square3/2(In2), square3/1(In1)
  delayMatch35/1 -> subtract6/1(In1)
  delayMatch26/1 -> adder7/1(In1)
  adder/1(Out1) -> J/1
  square/1(Out1) -> delayMatch21/1
  adder1/1(Out1) -> adder/1(In1)
  subtract/1(Out1) -> subtract_outbuff/1
  square1/1(Out1) -> delayMatch20/1
  adder2/1(Out1) -> adder1/1(In1)
  adder3/1(Out1) -> subtract/2(In2)
  subtract1/1(Out1) -> subtract_outbuff1/1
  square2/1(Out1) -> adder2/2(In2)
  square3/1(Out1) -> delayMatch49/1
  multiplier/1(Out1) -> adder3/1(In1)
  adder4/1(Out1) -> subtract1/2(In2)
  subtract2/1(Out1) -> subtract_outbuff2/1
  subtract3/1(Out1) -> subtract_outbuff3/1
  subtract4/1(Out1) -> multiplier/2(In2)
  multiplier1/1(Out1) -> adder4/1(In1)
  adder5/1(Out1) -> subtract2/2(In2)
  adder6/1(Out1) -> subtract3/2(In2)
  multiplier2/1(Out1) -> subtract4/2(In2)
  subtract5/1(Out1) -> multiplier1/2(In2)
  multiplier3/1(Out1) -> adder5/1(In1)
  multiplier4/1(Out1) -> adder6/1(In1)
  multiplier5/1(Out1) -> subtract5/2(In2)
  subtract6/1(Out1) -> multiplier3/2(In2)
  adder7/1(Out1) -> multiplier4/2(In2)
  multiplier6/1(Out1) -> subtract6/2(In2)
  subtract7/1(Out1) -> delayMatch8/1
  multiplier7/1(Out1) -> adder7/2(In2)
  subtract8/1(Out1) -> delayMatch26/1
  adder8/1(Out1) -> multiplier6/2(In2)
  multiplier8/1(Out1) -> subtract7/2(In2)
  multiplier9/1(Out1) -> multiplier7/1(In1)
  multiplier10/1(Out1) -> subtract8/2(In2)
  multiplier11/1(Out1) -> adder8/2(In2)
  delayMatch37/1 -> adder5/2(In2)
  delayMatch23/1 -> multiplier10/2(In2)
  delayMatch22/1 -> multiplier9/2(In2)
  delayMatch32/1 -> multiplier11/2(In2)
  delayMatch30/1 -> multiplier8/2(In2)
  delayMatch/1 -> delayMatch24/1
  delayMatch1/1 -> delayMatch25/1
  delayMatch2/1 -> delayMatch27/1
  delayMatch3/1 -> delayMatch28/1
  delayMatch4/1 -> delayMatch29/1
  delayMatch39/1 -> multiplier5/2(In2)
  delayMatch6/1 -> delayMatch31/1
  delayMatch5/1 -> delayMatch33/1
  delayMatch7/1 -> delayMatch34/1
  delayMatch8/1 -> delayMatch35/1
  delayMatch9/1 -> delayMatch36/1
  delayMatch10/1 -> delayMatch37/1
  delayMatch11/1 -> delayMatch38/1
  delayMatch44/1 -> multiplier2/2(In2)
  delayMatch12/1 -> delayMatch40/1
  delayMatch13/1 -> delayMatch41/1
  delayMatch14/1 -> delayMatch42/1
  delayMatch15/1 -> delayMatch43/1
  delayMatch16/1 -> delayMatch45/1
  delayMatch17/1 -> delayMatch46/1
  delayMatch18/1 -> delayMatch47/1
  delayMatch19/1 -> delayMatch48/1
  delayMatch20/1 -> delayMatch50/1
  delayMatch21/1 -> delayMatch51/1
  SampleTime_div_Ld/1 -> delayMatch2/1
  SampleTime_div_Lq/1 -> delayMatch9/1
  SampleTime_div_Lx/1 -> delayMatch13/1
  SampleTime_div_Ly/1 -> delayMatch17/1
  id_k_1/1 -> delayMatch3/1, multiplier11/1(In1), multiplier10/1(In1)
  iq_k_1/1 -> delayMatch10/1, delayMatch1/1, multiplier8/1(In1)
  ix_k_1/1 -> delayMatch14/1, multiplier5/1(In1)
  iy_k_1/1 -> delayMatch18/1, multiplier2/1(In1)
  Rs/1 -> delayMatch44/1, delayMatch39/1, delayMatch30/1, delayMatch23/1
  omega_el/1 -> delayMatch7/1, multiplier9/1(In1)
  Lq/1 -> delayMatch22/1
  Ld/1 -> delayMatch32/1
  psiPM/1 -> delayMatch5/1
  d_phase_voltage_per_switching_state/1 -> delayMatch/1
  q_phase_voltage_per_switching_state/1 -> delayMatch6/1
  x_phase_voltage_per_switching_state/1 -> delayMatch12/1
  y_phase_voltage_per_switching_state/1 -> delayMatch16/1
  id_ref/1 -> delayMatch4/1
  iq_ref/1 -> delayMatch11/1
  ix_ref/1 -> delayMatch15/1
  iy_ref/1 -> delayMatch19/1

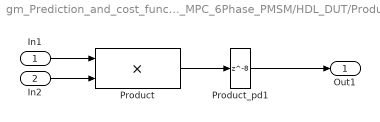
== system gm_Prediction_and_cost_function_FCS_MPC_6Phase_PMSM/HDL_DUT/Product ==
  In1 : Inport
  In2 : Inport  Port=2
  Product : Product  Inputs=**  OutDataTypeStr=single  SampleTime=1e-08
  Product_pd1 : Delay  DelayLength=8
  Out1 : Outport
  wires:
  In1/1 -> Product/1
  In2/1 -> Product/2
  Product/1 -> Product_pd1/1
  Product_pd1/1 -> Out1/1

== system gm_Prediction_and_cost_function_FCS_MPC_6Phase_PMSM/HDL_DUT/Detect Rise Positive/Positive ==
  u : Inport  OutDataTypeStr=boolean  SampleTime=1e-08
  Compare : RelationalOperator  Operator=>  OutDataTypeStr=boolean  ZeroCross=off
  Constant : Constant  DisableCoverage=on  Value=0  OutDataTypeStr=Inherit: Inherit via back propagation  SampleTime=-1  PreserveConstantTs=on
  y : Outport  SampleTime=1e-08
  wires:
  Compare/1 -> y/1
  Constant/1 -> Compare/2
  u/1 -> Compare/1

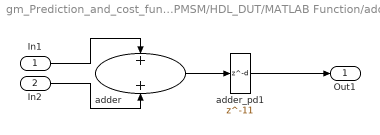
== system gm_Prediction_and_cost_function_FCS_MPC_6Phase_PMSM/HDL_DUT/MATLAB Function/adder ==
  In1 : Inport
  In2 : Inport  Port=2
  adder : Sum  OutDataTypeStr=single  SampleTime=1e-08
  adder_pd1 : Delay  DelayLength=11
  Out1 : Outport
  wires:
  In1/1 -> adder/1
  In2/1 -> adder/2
  adder/1 -> adder_pd1/1
  adder_pd1/1 -> Out1/1

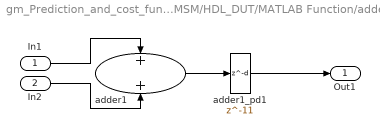
== system gm_Prediction_and_cost_function_FCS_MPC_6Phase_PMSM/HDL_DUT/MATLAB Function/adder1 ==
  In1 : Inport
  In2 : Inport  Port=2
  adder1 : Sum  OutDataTypeStr=single  SampleTime=1e-08
  adder1_pd1 : Delay  DelayLength=11
  Out1 : Outport
  wires:
  In1/1 -> adder1/1
  In2/1 -> adder1/2
  adder1/1 -> adder1_pd1/1
  adder1_pd1/1 -> Out1/1

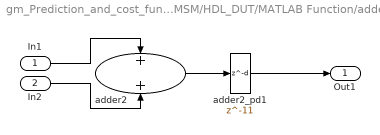
== system gm_Prediction_and_cost_function_FCS_MPC_6Phase_PMSM/HDL_DUT/MATLAB Function/adder2 ==
  In1 : Inport
  In2 : Inport  Port=2
  adder2 : Sum  OutDataTypeStr=single  SampleTime=1e-08
  adder2_pd1 : Delay  DelayLength=11
  Out1 : Outport
  wires:
  In1/1 -> adder2/1
  In2/1 -> adder2/2
  adder2/1 -> adder2_pd1/1
  adder2_pd1/1 -> Out1/1

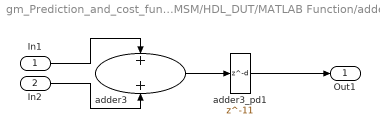
== system gm_Prediction_and_cost_function_FCS_MPC_6Phase_PMSM/HDL_DUT/MATLAB Function/adder3 ==
  In1 : Inport
  In2 : Inport  Port=2
  adder3 : Sum  OutDataTypeStr=single  SampleTime=1e-08
  adder3_pd1 : Delay  DelayLength=11
  Out1 : Outport
  wires:
  In1/1 -> adder3/1
  In2/1 -> adder3/2
  adder3/1 -> adder3_pd1/1
  adder3_pd1/1 -> Out1/1

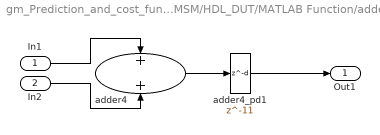
== system gm_Prediction_and_cost_function_FCS_MPC_6Phase_PMSM/HDL_DUT/MATLAB Function/adder4 ==
  In1 : Inport
  In2 : Inport  Port=2
  adder4 : Sum  OutDataTypeStr=single  SampleTime=1e-08
  adder4_pd1 : Delay  DelayLength=11
  Out1 : Outport
  wires:
  In1/1 -> adder4/1
  In2/1 -> adder4/2
  adder4/1 -> adder4_pd1/1
  adder4_pd1/1 -> Out1/1

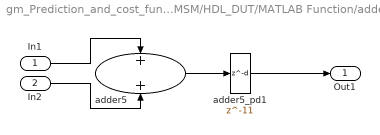
== system gm_Prediction_and_cost_function_FCS_MPC_6Phase_PMSM/HDL_DUT/MATLAB Function/adder5 ==
  In1 : Inport
  In2 : Inport  Port=2
  adder5 : Sum  OutDataTypeStr=single  SampleTime=1e-08
  adder5_pd1 : Delay  DelayLength=11
  Out1 : Outport
  wires:
  In1/1 -> adder5/1
  In2/1 -> adder5/2
  adder5/1 -> adder5_pd1/1
  adder5_pd1/1 -> Out1/1

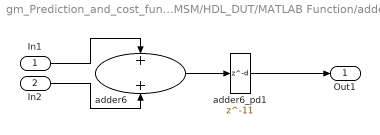
== system gm_Prediction_and_cost_function_FCS_MPC_6Phase_PMSM/HDL_DUT/MATLAB Function/adder6 ==
  In1 : Inport
  In2 : Inport  Port=2
  adder6 : Sum  OutDataTypeStr=single  SampleTime=1e-08
  adder6_pd1 : Delay  DelayLength=11
  Out1 : Outport
  wires:
  In1/1 -> adder6/1
  In2/1 -> adder6/2
  adder6/1 -> adder6_pd1/1
  adder6_pd1/1 -> Out1/1

== system gm_Prediction_and_cost_function_FCS_MPC_6Phase_PMSM/HDL_DUT/MATLAB Function/adder7 ==
  In1 : Inport
  In2 : Inport  Port=2
  adder7 : Sum  OutDataTypeStr=single  SampleTime=1e-08
  adder7_pd1 : Delay  DelayLength=11
  Out1 : Outport
  wires:
  In1/1 -> adder7/1
  In2/1 -> adder7/2
  adder7/1 -> adder7_pd1/1
  adder7_pd1/1 -> Out1/1

== system gm_Prediction_and_cost_function_FCS_MPC_6Phase_PMSM/HDL_DUT/MATLAB Function/adder8 ==
  In1 : Inport
  In2 : Inport  Port=2
  adder8 : Sum  OutDataTypeStr=single  SampleTime=1e-08
  adder8_pd1 : Delay  DelayLength=11
  Out1 : Outport
  wires:
  In1/1 -> adder8/1
  In2/1 -> adder8/2
  adder8/1 -> adder8_pd1/1
  adder8_pd1/1 -> Out1/1

== system gm_Prediction_and_cost_function_FCS_MPC_6Phase_PMSM/HDL_DUT/MATLAB Function/multiplier ==
  In1 : Inport
  In2 : Inport  Port=2
  multiplier : Product  Inputs=**  OutDataTypeStr=single  SampleTime=1e-08
  multiplier_pd1 : Delay  DelayLength=8
  Out1 : Outport
  wires:
  In1/1 -> multiplier/1
  In2/1 -> multiplier/2
  multiplier/1 -> multiplier_pd1/1
  multiplier_pd1/1 -> Out1/1

== system gm_Prediction_and_cost_function_FCS_MPC_6Phase_PMSM/HDL_DUT/MATLAB Function/multiplier1 ==
  In1 : Inport
  In2 : Inport  Port=2
  multiplier1 : Product  Inputs=**  OutDataTypeStr=single  SampleTime=1e-08
  multiplier1_pd1 : Delay  DelayLength=8
  Out1 : Outport
  wires:
  In1/1 -> multiplier1/1
  In2/1 -> multiplier1/2
  multiplier1/1 -> multiplier1_pd1/1
  multiplier1_pd1/1 -> Out1/1

== system gm_Prediction_and_cost_function_FCS_MPC_6Phase_PMSM/HDL_DUT/MATLAB Function/multiplier10 ==
  In1 : Inport
  In2 : Inport  Port=2
  multiplier10 : Product  Inputs=**  OutDataTypeStr=single  SampleTime=1e-08
  multiplier10_pd1 : Delay  DelayLength=8
  Out1 : Outport
  wires:
  In1/1 -> multiplier10/1
  In2/1 -> multiplier10/2
  multiplier10/1 -> multiplier10_pd1/1
  multiplier10_pd1/1 -> Out1/1

== system gm_Prediction_and_cost_function_FCS_MPC_6Phase_PMSM/HDL_DUT/MATLAB Function/multiplier11 ==
  In1 : Inport
  In2 : Inport  Port=2
  multiplier11 : Product  Inputs=**  OutDataTypeStr=single  SampleTime=1e-08
  multiplier11_pd1 : Delay  DelayLength=8
  Out1 : Outport
  wires:
  In1/1 -> multiplier11/1
  In2/1 -> multiplier11/2
  multiplier11/1 -> multiplier11_pd1/1
  multiplier11_pd1/1 -> Out1/1

== system gm_Prediction_and_cost_function_FCS_MPC_6Phase_PMSM/HDL_DUT/MATLAB Function/multiplier2 ==
  In1 : Inport
  In2 : Inport  Port=2
  multiplier2 : Product  Inputs=**  OutDataTypeStr=single  SampleTime=1e-08
  multiplier2_pd1 : Delay  DelayLength=8
  Out1 : Outport
  wires:
  In1/1 -> multiplier2/1
  In2/1 -> multiplier2/2
  multiplier2/1 -> multiplier2_pd1/1
  multiplier2_pd1/1 -> Out1/1

== system gm_Prediction_and_cost_function_FCS_MPC_6Phase_PMSM/HDL_DUT/MATLAB Function/multiplier3 ==
  In1 : Inport
  In2 : Inport  Port=2
  multiplier3 : Product  Inputs=**  OutDataTypeStr=single  SampleTime=1e-08
  multiplier3_pd1 : Delay  DelayLength=8
  Out1 : Outport
  wires:
  In1/1 -> multiplier3/1
  In2/1 -> multiplier3/2
  multiplier3/1 -> multiplier3_pd1/1
  multiplier3_pd1/1 -> Out1/1

== system gm_Prediction_and_cost_function_FCS_MPC_6Phase_PMSM/HDL_DUT/MATLAB Function/multiplier4 ==
  In1 : Inport
  In2 : Inport  Port=2
  multiplier4 : Product  Inputs=**  OutDataTypeStr=single  SampleTime=1e-08
  multiplier4_pd1 : Delay  DelayLength=8
  Out1 : Outport
  wires:
  In1/1 -> multiplier4/1
  In2/1 -> multiplier4/2
  multiplier4/1 -> multiplier4_pd1/1
  multiplier4_pd1/1 -> Out1/1

== system gm_Prediction_and_cost_function_FCS_MPC_6Phase_PMSM/HDL_DUT/MATLAB Function/multiplier5 ==
  In1 : Inport
  In2 : Inport  Port=2
  multiplier5 : Product  Inputs=**  OutDataTypeStr=single  SampleTime=1e-08
  multiplier5_pd1 : Delay  DelayLength=8
  Out1 : Outport
  wires:
  In1/1 -> multiplier5/1
  In2/1 -> multiplier5/2
  multiplier5/1 -> multiplier5_pd1/1
  multiplier5_pd1/1 -> Out1/1

== system gm_Prediction_and_cost_function_FCS_MPC_6Phase_PMSM/HDL_DUT/MATLAB Function/multiplier6 ==
  In1 : Inport
  In2 : Inport  Port=2
  multiplier6 : Product  Inputs=**  OutDataTypeStr=single  SampleTime=1e-08
  multiplier6_pd1 : Delay  DelayLength=8
  Out1 : Outport
  wires:
  In1/1 -> multiplier6/1
  In2/1 -> multiplier6/2
  multiplier6/1 -> multiplier6_pd1/1
  multiplier6_pd1/1 -> Out1/1

== system gm_Prediction_and_cost_function_FCS_MPC_6Phase_PMSM/HDL_DUT/MATLAB Function/multiplier7 ==
  In1 : Inport
  In2 : Inport  Port=2
  multiplier7 : Product  Inputs=**  OutDataTypeStr=single  SampleTime=1e-08
  multiplier7_pd1 : Delay  DelayLength=8
  Out1 : Outport
  wires:
  In1/1 -> multiplier7/1
  In2/1 -> multiplier7/2
  multiplier7/1 -> multiplier7_pd1/1
  multiplier7_pd1/1 -> Out1/1

== system gm_Prediction_and_cost_function_FCS_MPC_6Phase_PMSM/HDL_DUT/MATLAB Function/multiplier8 ==
  In1 : Inport
  In2 : Inport  Port=2
  multiplier8 : Product  Inputs=**  OutDataTypeStr=single  SampleTime=1e-08
  multiplier8_pd1 : Delay  DelayLength=8
  Out1 : Outport
  wires:
  In1/1 -> multiplier8/1
  In2/1 -> multiplier8/2
  multiplier8/1 -> multiplier8_pd1/1
  multiplier8_pd1/1 -> Out1/1

== system gm_Prediction_and_cost_function_FCS_MPC_6Phase_PMSM/HDL_DUT/MATLAB Function/multiplier9 ==
  In1 : Inport
  In2 : Inport  Port=2
  multiplier9 : Product  Inputs=**  OutDataTypeStr=single  SampleTime=1e-08
  multiplier9_pd1 : Delay  DelayLength=8
  Out1 : Outport
  wires:
  In1/1 -> multiplier9/1
  In2/1 -> multiplier9/2
  multiplier9/1 -> multiplier9_pd1/1
  multiplier9_pd1/1 -> Out1/1

== system gm_Prediction_and_cost_function_FCS_MPC_6Phase_PMSM/HDL_DUT/MATLAB Function/square ==
  In1 : Inport
  In2 : Inport  Port=2
  square : Product  Inputs=**  OutDataTypeStr=single  SampleTime=1e-08
  square_pd1 : Delay  DelayLength=8
  Out1 : Outport
  wires:
  In1/1 -> square/1
  In2/1 -> square/2
  square/1 -> square_pd1/1
  square_pd1/1 -> Out1/1

== system gm_Prediction_and_cost_function_FCS_MPC_6Phase_PMSM/HDL_DUT/MATLAB Function/square1 ==
  In1 : Inport
  In2 : Inport  Port=2
  square1 : Product  Inputs=**  OutDataTypeStr=single  SampleTime=1e-08
  square1_pd1 : Delay  DelayLength=8
  Out1 : Outport
  wires:
  In1/1 -> square1/1
  In2/1 -> square1/2
  square1/1 -> square1_pd1/1
  square1_pd1/1 -> Out1/1

== system gm_Prediction_and_cost_function_FCS_MPC_6Phase_PMSM/HDL_DUT/MATLAB Function/square2 ==
  In1 : Inport
  In2 : Inport  Port=2
  square2 : Product  Inputs=**  OutDataTypeStr=single  SampleTime=1e-08
  square2_pd1 : Delay  DelayLength=8
  Out1 : Outport
  wires:
  In1/1 -> square2/1
  In2/1 -> square2/2
  square2/1 -> square2_pd1/1
  square2_pd1/1 -> Out1/1
